simulink model "estimate_battery_soca"  (R2022a)
settings: Solver=VariableStepAuto  StartTime=0.0  StopTime=t_end  RelTol=1e-3
values from neighbouring files (symbols this model uses):
  Bat_cap = 1.241    [eba_const_setting.m]
  eff_bcr = 80    [eba_const_setting.m]
  eff_id = 90    [eba_const_setting.m]
  eff_pcm = 90    [eba_const_setting.m]
  eff_tmp = 90    [eba_const_setting.m]
  Np = 4    [eba_const_setting.m]
  Ns = 2    [eba_const_setting.m]
  OCV = [3 ... (first row only)    [eba_const_setting.m]
  Ri_cell = (140+190)/2*1e-3    (= 0.165)    [eba_const_setting.m]
  SOC = [0:5:100]    [new_power_generation_model_alpha_0.m]    (also in new_power_generation_model_alpha_0_EO.m; new_power_generation_model_alpha_0_mission.m; new_power_generation_model_alpha_1.m; new_power_generation_model_alpha_1_EO.m)
  SOC_init = SOC0/100    [new_power_generation_model_alpha_0.m]    (also in new_power_generation_model_alpha_0_EO.m; new_power_generation_model_alpha_0_mission.m; new_power_generation_model_alpha_1.m; new_power_generation_model_alpha_1_EO.m)
  V_ulim = 8.26    [eba_const_setting.m]
undefined symbols (not defined in the file or in its folder): sigbuilder_block
settings Model: Creator=Geuk-Nam Kim  LastModifiedBy=ACL2022_13
settings SolverCC: ZeroCrossAlgorithm=Adaptive  AlgebraicLoopSolver=TrustRegion
settings DebuggingCC: IgnoredZcDiagnostic=none  UnconnectedInputMsg=warning  UnconnectedOutputMsg=warning  UnconnectedLineMsg=warning  SFMachineParentedDataDiag=warning

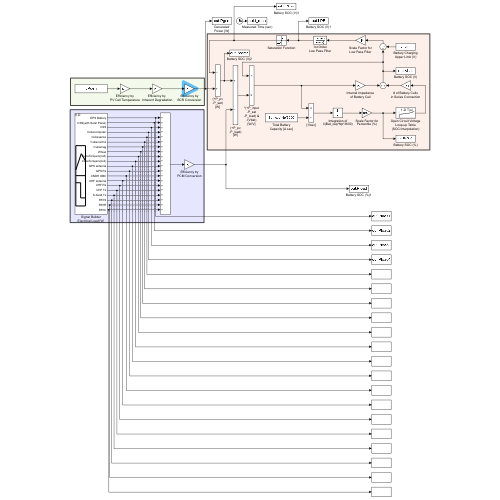
[thumbnail: Simulink's stored preview of the top-level diagram]
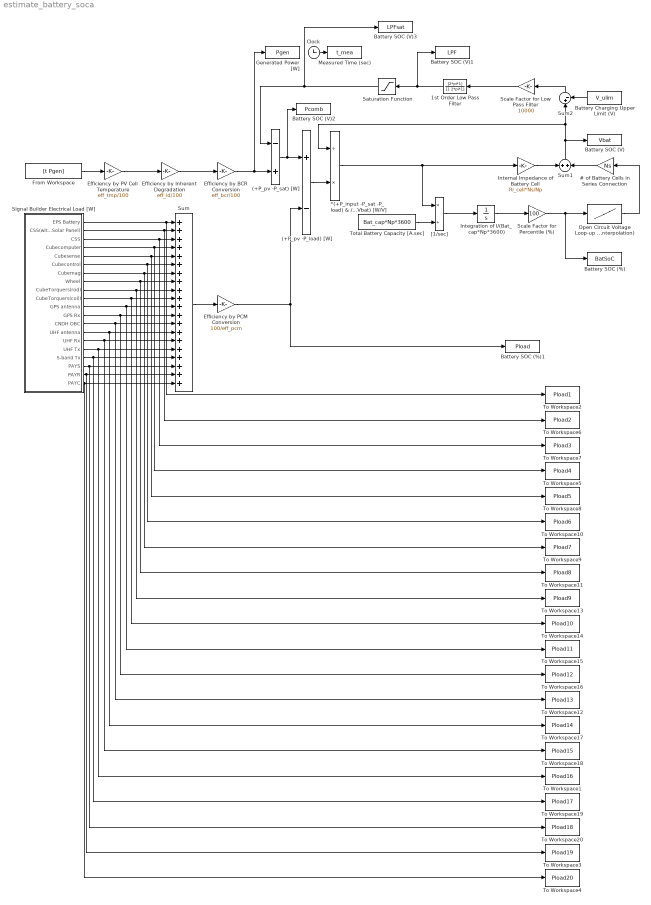
== system estimate_battery_soca ==
  # of Battery Cells in Series Connection : Gain  Gain=Ns
  (+P_pv -P_load) [W] : Sum  Inputs=+-
  (+P_pv -P_sat) [W] : Sum  Inputs=-+
  *(+P_input -P_sat -P_load) & /(Vbat) [W/V] : Product  Inputs=/*
  1st Order Low Pass Filter : TransferFcn  Numerator=[2*pi*1]  Denominator=[1 2*pi*1]
  Battery Charging Upper Limit (V) : Constant  Value=V_ulim
  Battery SOC (%) : ToWorkspace  VariableName=BatSoC  SampleTime=-1
  Battery SOC (%)1 : ToWorkspace  VariableName=Pload  SampleTime=-1
  Battery SOC (V) : ToWorkspace  VariableName=Vbat  SampleTime=-1
  Battery SOC (V)1 : ToWorkspace  VariableName=LPF  SampleTime=-1
  Battery SOC (V)2 : ToWorkspace  VariableName=Pcomb  SampleTime=-1
  Battery SOC (V)3 : ToWorkspace  VariableName=LPFsat  SampleTime=-1
  Clock : Clock
  "Efficiency by BCR Conversion " : Gain  Gain=eff_bcr/100
  Efficiency by PCM Conversion : Gain  Gain=100/eff_pcm
  Efficiency by PV Cell Temperature : Gain  Gain=eff_tmp/100
  Efficiency by Inherent Degradation : Gain  Gain=eff_id/100
  From Workspace : FromWorkspace  VariableName=[t Pgen]  SampleTime=-1
  Generated Power [W] : ToWorkspace  VariableName=Pgen  SampleTime=-1
  Integration of I/(Bat_cap*Np*3600) : Integrator  InitialCondition=SOC_init
  Internal Impedance of Battery Cell : Gain  Gain=Ri_cell*Ns/Np
  Measured Time (sec) : ToWorkspace  VariableName=t_mea  SampleTime=-1
  Open Circuit Voltage Loop-up Table (SOC Interpolation) : Lookup_n-D  NumberOfTableDimensions=1  BreakpointsForDimension1=SOC  Table=OCV  InternalRulePriority=Speed  RndMeth=Simplest
  Saturation Function : Saturate  UpperLimit=V_ulim  LowerLimit=0
  Scale Factor for Low Pass Filter : Gain  Gain=10000
  Scale Factor for Percentile (%) : Gain  Gain=100
  Signal Builder Electrical Load [W] : Subsystem  Tag=STV Subsys  LoadFcn=sigbuilder_block('load');  StartFcn=sigbuilder_block('start');  StopFcn=sigbuilder_block('stop');  ClipboardFcn=sigbuilder_block('clipboard');  mask(Sigbuilder block){tuvar=[0:10]}
      mask help: Simulink:masks:SigbuilderBlock_MD
      mask init:
      | if ~strcmp(get_param(bdroot(gcbh),'SimulationStatus'),'stopped') tuvar = sigbuilder_block('maskInit'); end
      settings: CopyFcn=sigbuilder_block('copy');  DeleteFcn=sigbuilder_block('delete');  ModelCloseFcn=sigbuilder_block('modelClose');  PreSaveFcn=sigbuilder_block('preSave');  PauseFcn=sigbuilder_block('pause');  ContinueFcn=sigbuilder_block('continue');  NameChangeFcn=sigbuilder_block('namechange');  OpenFcn=sigbuilder_block('open',[6 30 1428 680.25 ]);  CloseFcn=sigbuilder_block('close');
      mask Display: plot(0, 0, 100, 100,[2, 2, 32, 32, 2], [68, 8, 8, 68, 68],[32, 2], [38, 38], [32, 19, 2],[53, 60, 44], [32, 17, 17, 2],[16, 16, 31, 31]);txt = getActiveGroup(gcbh);text(2, 100, txt,'verticalAlignment', 'top');
  Sum : Sum  Inputs=20
  Sum1 : Sum  Inputs=+|+
  Sum2 : Sum  Inputs=|+-
  To Workspace1 : ToWorkspace  VariableName=Pload16  SampleTime=-1
  To Workspace10 : ToWorkspace  VariableName=Pload6  SampleTime=-1
  To Workspace11 : ToWorkspace  VariableName=Pload8  SampleTime=-1
  To Workspace12 : ToWorkspace  VariableName=Pload13  SampleTime=-1
  To Workspace13 : ToWorkspace  VariableName=Pload9  SampleTime=-1
  To Workspace14 : ToWorkspace  VariableName=Pload10  SampleTime=-1
  To Workspace15 : ToWorkspace  VariableName=Pload11  SampleTime=-1
  To Workspace16 : ToWorkspace  VariableName=Pload12  SampleTime=-1
  To Workspace17 : ToWorkspace  VariableName=Pload14  SampleTime=-1
  To Workspace18 : ToWorkspace  VariableName=Pload15  SampleTime=-1
  To Workspace19 : ToWorkspace  VariableName=Pload17  SampleTime=-1
  To Workspace2 : ToWorkspace  VariableName=Pload1  SampleTime=-1
  To Workspace20 : ToWorkspace  VariableName=Pload18  SampleTime=-1
  To Workspace3 : ToWorkspace  VariableName=Pload19  SampleTime=-1
  To Workspace4 : ToWorkspace  VariableName=Pload20  SampleTime=-1
  To Workspace5 : ToWorkspace  VariableName=Pload4  SampleTime=-1
  To Workspace6 : ToWorkspace  VariableName=Pload2  SampleTime=-1
  To Workspace7 : ToWorkspace  VariableName=Pload3  SampleTime=-1
  To Workspace8 : ToWorkspace  VariableName=Pload5  SampleTime=-1
  To Workspace9 : ToWorkspace  VariableName=Pload7  SampleTime=-1
  Total Battery Capacity [A.sec] : Constant  Value=Bat_cap*Np*3600
  "[1/sec]" : Product  Inputs=*/
  wires:
  From Workspace/1 -> Efficiency by PV Cell Temperature/1
  Open Circuit Voltage Loop-up Table (SOC Interpolation)/1 -> # of Battery Cells in Series Connection/1
  Signal Builder Electrical Load [W]/8(Wheel) -> To Workspace11/1, Sum/8
  Total Battery Capacity [A.sec]/1 -> "[1/sec]"/2
  Sum2/1 -> Scale Factor for Low Pass Filter/1
  "[1/sec]"/1 -> Integration of I/(Bat_cap*Np*3600)/1
  Scale Factor for Percentile (%)/1 -> Battery SOC (%)/1, Open Circuit Voltage Loop-up Table (SOC Interpolation)/1
  Signal Builder Electrical Load [W]/1(EPS Battery) -> To Workspace2/1, Sum/1
  "Efficiency by BCR Conversion "/1 -> (+P_pv -P_sat) [W]/2, Generated Power [W]/1
  Signal Builder Electrical Load [W]/14(UHF antenna) -> To Workspace17/1, Sum/14
  # of Battery Cells in Series Connection/1 -> Sum1/2
  Signal Builder Electrical Load [W]/4(Cubecomputer) -> To Workspace5/1, Sum/4
  Integration of I/(Bat_cap*Np*3600)/1 -> Scale Factor for Percentile (%)/1
  *(+P_input -P_sat -P_load) & /(Vbat) [W/V]/1 -> "[1/sec]"/1, Internal Impedance of Battery Cell/1
  Internal Impedance of Battery Cell/1 -> Sum1/1
  1st Order Low Pass Filter/1 -> Battery SOC (V)1/1, Saturation Function/1
  Signal Builder Electrical Load [W]/12(GPS Rx) -> To Workspace16/1, Sum/12
  Signal Builder Electrical Load [W]/13(CNDH OBC) -> To Workspace12/1, Sum/13
  Saturation Function/1 -> Battery SOC (V)3/1, (+P_pv -P_sat) [W]/1
  Signal Builder Electrical Load [W]/10(CubeTorquers(coil)) -> To Workspace14/1, Sum/10
  (+P_pv -P_load) [W]/1 -> *(+P_input -P_sat -P_load) & /(Vbat) [W/V]/2
  Signal Builder Electrical Load [W]/11(GPS antenna) -> To Workspace15/1, Sum/11
  Signal Builder Electrical Load [W]/2(CSS(with Solar Panel)) -> To Workspace6/1, Sum/2
  Battery Charging Upper Limit (V)/1 -> Sum2/2
  Signal Builder Electrical Load [W]/15(UHF Rx) -> To Workspace18/1, Sum/15
  Signal Builder Electrical Load [W]/6(Cubecontrol) -> To Workspace10/1, Sum/6
  Sum1/1 -> Sum2/1, *(+P_input -P_sat -P_load) & /(Vbat) [W/V]/1, Battery SOC (V)/1
  Signal Builder Electrical Load [W]/5(Cubesense) -> To Workspace8/1, Sum/5
  Signal Builder Electrical Load [W]/9(CubeTorquers(rod)) -> To Workspace13/1, Sum/9
  Clock/1 -> Measured Time (sec)/1
  Efficiency by Inherent Degradation/1 -> "Efficiency by BCR Conversion "/1
  Sum/1 -> Efficiency by PCM Conversion/1
  Signal Builder Electrical Load [W]/3(CSS) -> To Workspace7/1, Sum/3
  Efficiency by PV Cell Temperature/1 -> Efficiency by Inherent Degradation/1
  Signal Builder Electrical Load [W]/7(Cubemag) -> To Workspace9/1, Sum/7
  (+P_pv -P_sat) [W]/1 -> Battery SOC (V)2/1, (+P_pv -P_load) [W]/1
  Scale Factor for Low Pass Filter/1 -> 1st Order Low Pass Filter/1
  Efficiency by PCM Conversion/1 -> (+P_pv -P_load) [W]/2, Battery SOC (%)1/1
  Signal Builder Electrical Load [W]/16(UHF Tx) -> To Workspace1/1, Sum/16
  Signal Builder Electrical Load [W]/17(S-band Tx) -> To Workspace19/1, Sum/17
  Signal Builder Electrical Load [W]/18(PAYS) -> To Workspace20/1, Sum/18
  Signal Builder Electrical Load [W]/19(PAYR) -> To Workspace3/1, Sum/19
  Signal Builder Electrical Load [W]/20(PAYC) -> To Workspace4/1, Sum/20

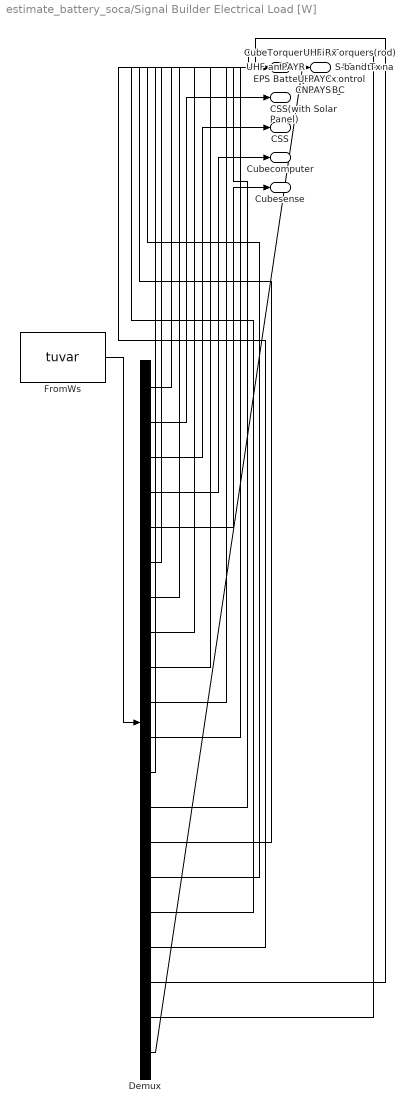
== system estimate_battery_soca/Signal Builder Electrical Load [W] ==
  Demux : Demux  Tag=STV Demux  Outputs=20
      settings: DisplayOption=none
  FromWs : FromWorkspace  Tag=STV FromWs  VariableName=tuvar
  EPS Battery : Outport  VectorParamsAs1DForOutWhenUnconnected=off
  CSS(with Solar Panel) : Outport  Tag=STV Outport  Port=2  VectorParamsAs1DForOutWhenUnconnected=off
  CSS : Outport  Tag=STV Outport  Port=3  VectorParamsAs1DForOutWhenUnconnected=off
  Cubecomputer : Outport  Tag=STV Outport  Port=4  VectorParamsAs1DForOutWhenUnconnected=off
  Cubesense : Outport  Tag=STV Outport  Port=5  VectorParamsAs1DForOutWhenUnconnected=off
  Cubecontrol : Outport  Tag=STV Outport  Port=6  VectorParamsAs1DForOutWhenUnconnected=off
  Cubemag : Outport  Tag=STV Outport  Port=7  VectorParamsAs1DForOutWhenUnconnected=off
  Wheel : Outport  Tag=STV Outport  Port=8  VectorParamsAs1DForOutWhenUnconnected=off
  CubeTorquers(rod) : Outport  Tag=STV Outport  Port=9  VectorParamsAs1DForOutWhenUnconnected=off
  CubeTorquers(coil) : Outport  Tag=STV Outport  Port=10  VectorParamsAs1DForOutWhenUnconnected=off
  GPS antenna : Outport  Tag=STV Outport  Port=11  VectorParamsAs1DForOutWhenUnconnected=off
  GPS Rx : Outport  Tag=STV Outport  Port=12  VectorParamsAs1DForOutWhenUnconnected=off
  CNDH OBC : Outport  Tag=STV Outport  Port=13
  UHF antenna : Outport  Tag=STV Outport  Port=14
  UHF Rx : Outport  Tag=STV Outport  Port=15
  UHF Tx : Outport  Tag=STV Outport  Port=16
  S-band Tx : Outport  Tag=STV Outport  Port=17
  PAYS : Outport  Tag=STV Outport  Port=18
  PAYR : Outport  Tag=STV Outport  Port=19
  PAYC : Outport  Tag=STV Outport  Port=20
  wires:
  Demux/1 -> EPS Battery/1
  Demux/2 -> CSS(with Solar Panel)/1
  Demux/3 -> CSS/1
  Demux/4 -> Cubecomputer/1
  Demux/5 -> Cubesense/1
  Demux/6 -> Cubecontrol/1
  Demux/7 -> Cubemag/1
  FromWs/1 -> Demux/1
  Demux/8 -> Wheel/1
  Demux/9 -> CubeTorquers(rod)/1
  Demux/10 -> CubeTorquers(coil)/1
  Demux/11 -> GPS antenna/1
  Demux/12 -> GPS Rx/1
  Demux/13 -> CNDH OBC/1
  Demux/14 -> UHF antenna/1
  Demux/15 -> UHF Rx/1
  Demux/16 -> UHF Tx/1
  Demux/17 -> S-band Tx/1
  Demux/18 -> PAYS/1
  Demux/19 -> PAYR/1
  Demux/20 -> PAYC/1
